simulink model "model"  (R2021a)
settings: Solver=FixedStepAuto  StartTime=0  StopTime=inf  FixedStep=inits.dt  RelTol=1e-3
values from neighbouring files (symbols this model uses):
  inits = load('data.mat')    [main.m]
libraries: aerolibasang x3, shared6dof x1, aerolibatmos2 x1
settings Model: PauseTimes=0.1  Creator=Alper  LastModifiedBy=Alper

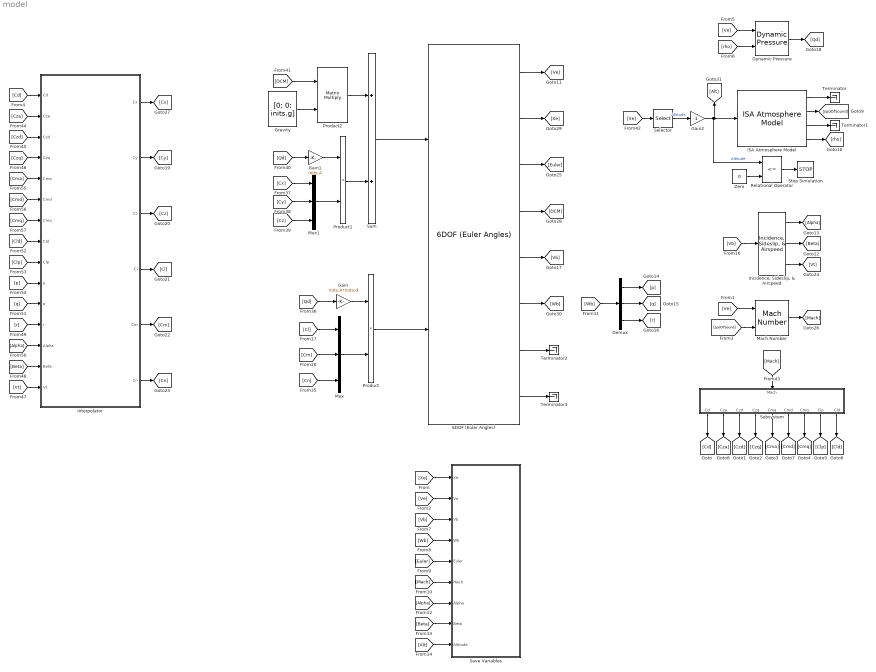
== system model ==
  6DOF (Euler Angles) : shared6dof/6DOF (Euler Angles)  units=Metric (MKS)  mtype=Fixed  rep=Euler Angles  xme_0=[inits.xm inits.ym inits.zm]  Vm_0=[inits.uInit inits.vInit inits.wInit]  eul_0=[inits.phiInit inits.thetaInit inits.psiInit]  pm_0=[inits.pInit inits.qInit inits.rInit]  mass_0=inits.m  mass_e=0.5  mass_f=2.0  inertia=inits.I  inertia_e=eye(3)  inertia_f=2*eye(3)  k_quat=1.0  vre_flag=on  abi_flag=off  aMode=0  xme_statename=''  Vm_statename=''  eul_statename=''  quat_statename=''  pm_statename=''  mass_statename=''
      settings: SourceProductBaseCode=AE,PW,DR,MT,UV,VE
  Demux : Demux  Outputs=3,
  Dynamic Pressure : aerolibasang/Dynamic Pressure
  Gain : Gain  Gain=inits.A*inits.d
  Gain1 : Gain  Gain=inits.A
  Gain2 : Gain  Gain=-1
  Gravity : Constant  Value=[0; 0; inits.g]  VectorParams1D=off
  ISA Atmosphere Model : aerolibatmos2/ISA Atmosphere Model  custom=off  g=9.80665  gamma=1.4  R=287.0531  L=0.0065  h_trop=11000  h_strat=20000  rho0=1.225  P0=101325  T0=288.15  h0=0
  "Incidence, Sideslip, & Airspeed" : aerolibasang/Incidence, Sideslip, & Airspeed
  Interpolator : Subsystem
  Mach Number : aerolibasang/Mach Number
      settings: SourceProductBaseCode=AE
  Mux : Mux  Inputs=3
  Mux1 : Mux  Inputs=3
  Product : Product
  Product1 : Product
  Product2 : Product  Multiplication=Matrix(*)
  Relational Operator : RelationalOperator  Operator=<=  OutDataTypeStr=boolean  RndMeth=Simplest
  Save Variables : Subsystem
  Selector : Selector  InputPortWidth=3  IndexOptions=Index vector (dialog)  Indices=3  OutputSizes=1
  Stop Simulation : Stop
  Subsystem : Subsystem
  Sum : Sum
  Terminator{,1..3} (4 alike) : Terminator
  Zero : Constant  Value=0  OutDataTypeStr=Inherit: Inherit via back propagation
  wires:
  Gain2/1 -> [Alt], ISA Atmosphere Model/1, Relational Operator/1  "Altitude"
  Subsystem/1(Cd) -> [Cd]
  Subsystem/2(Cza) -> [Cza]
  Subsystem/3(Czd) -> [Czd]
  Subsystem/4(Czq) -> [Czq]
  Subsystem/5(Cma) -> [Cma]
  Subsystem/6(Cmd) -> [Cmd]
  Subsystem/7(Cmq) -> [Cmq]
  Subsystem/8(Clp) -> [Clp]
  Subsystem/9(Cld) -> [Cld]
  ISA Atmosphere Model/2 -> [spdOfSound]
  ISA Atmosphere Model/4 -> [rho]
  "Incidence, Sideslip, & Airspeed"/2 -> [Beta]
  "Incidence, Sideslip, & Airspeed"/1 -> [Alpha]
  [Ve] -> Dynamic Pressure/1
  [rho] -> Dynamic Pressure/2
  Demux/1 -> [p]
  Demux/2 -> [q]
  Demux/3 -> [r]
  6DOF (Euler Angles)/1 -> [Ve]
  6DOF (Euler Angles)/5 -> [Vb]
  [Vb] -> "Incidence, Sideslip, & Airspeed"/1
  [spdOfSound] -> Mach Number/2
  [Ve] -> Mach Number/1
  Dynamic Pressure/1 -> [Qd]
  "Incidence, Sideslip, & Airspeed"/3 -> [Vt]
  6DOF (Euler Angles)/3 -> [Euler]
  [Cl] -> Mux/1
  [Cm] -> Mux/2
  [Cn] -> Mux/3
  [Qd] -> Gain/1
  Gain/1 -> Product/1
  Mux/1 -> Product/2
  Product/1 -> 6DOF (Euler Angles)/2
  6DOF (Euler Angles)/4 -> [DCM]
  [Cz] -> Mux1/3
  [Cy] -> Mux1/2
  Product1/1 -> Sum/2
  [Qd] -> Gain1/1
  [Cx] -> Mux1/1
  Gain1/1 -> Product1/1
  Mux1/1 -> Product1/2
  Gravity/1 -> Product2/2
  [DCM] -> Product2/1
  Product2/1 -> Sum/1
  Sum/1 -> 6DOF (Euler Angles)/1
  6DOF (Euler Angles)/2 -> [Xe]
  Zero/1 -> Relational Operator/2
  Relational Operator/1 -> Stop Simulation/1
  Mach Number/1 -> [Mach]
  [Mach] -> Subsystem/1(Mach)
  Interpolator/4(Cl) -> [Cl]
  Interpolator/3(Cz) -> [Cz]
  Interpolator/2(Cy) -> [Cy]
  Interpolator/1(Cx) -> [Cx]
  Interpolator/5(Cm) -> [Cm]
  Interpolator/6(Cn) -> [Cn]
  [Cd] -> Interpolator/1(Cd)
  [Cza] -> Interpolator/2(Cza)
  [Czd] -> Interpolator/3(Czd)
  [Czq] -> Interpolator/4(Czq)
  [Cma] -> Interpolator/5(Cma)
  [Cmd] -> Interpolator/6(Cmd)
  [Cmq] -> Interpolator/7(Cmq)
  [Cld] -> Interpolator/8(Cld)
  [Clp] -> Interpolator/9(Clp)
  [p] -> Interpolator/10(p)
  [q] -> Interpolator/11(q)
  [r] -> Interpolator/12(r)
  [Alpha] -> Interpolator/13(Alpha)
  [Beta] -> Interpolator/14(Beta)
  [Vt] -> Interpolator/15(Vt)
  6DOF (Euler Angles)/6 -> [Wb]
  [Wb] -> Demux/1
  [Xe] -> Save Variables/1(Xe)
  [Ve] -> Save Variables/2(Ve)
  [Vb] -> Save Variables/3(Vb)
  [Wb] -> Save Variables/4(Wb)
  [Euler] -> Save Variables/5(Euler)
  [Mach] -> Save Variables/6(Mach)
  [Alpha] -> Save Variables/7(Alpha)
  [Beta] -> Save Variables/8(Beta)
  [Xe] -> Selector/1
  Selector/1 -> Gain2/1  "Altitude"
  [Alt] -> Save Variables/9(Altitude)
  ISA Atmosphere Model/3 -> Terminator1/1
  ISA Atmosphere Model/1 -> Terminator/1
  6DOF (Euler Angles)/7 -> Terminator2/1
  6DOF (Euler Angles)/8 -> Terminator3/1

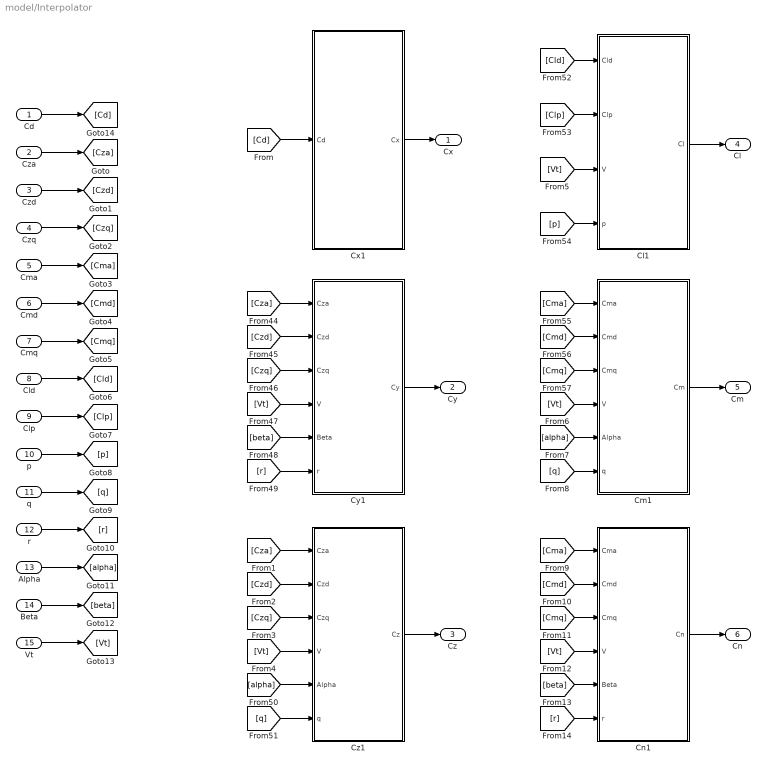
== system model/Interpolator ==
  Cd : Inport
  Cza : Inport  Port=2
  Czd : Inport  Port=3
  Czq : Inport  Port=4
  Cma : Inport  Port=5
  Cmd : Inport  Port=6
  Cmq : Inport  Port=7
  Cld : Inport  Port=8
  Clp : Inport  Port=9
  p : Inport  Port=10
  q : Inport  Port=11
  r : Inport  Port=12
  Alpha : Inport  Port=13
  Beta : Inport  Port=14
  Vt : Inport  Port=15
  Cl1 : Subsystem
  Cm1 : Subsystem
  Cn1 : Subsystem
  Cx1 : Subsystem
  Cy1 : Subsystem
  Cz1 : Subsystem
  Cx : Outport
  Cy : Outport  Port=2
  Cz : Outport  Port=3
  Cl : Outport  Port=4
  Cm : Outport  Port=5
  Cn : Outport  Port=6
  wires:
  Cz1/1(Cz) -> Cz/1
  Cy1/1(Cy) -> Cy/1
  Cl1/1(Cl) -> Cl/1
  Cn1/1(Cn) -> Cn/1
  Cm1/1(Cm) -> Cm/1
  Cza/1 -> [Cza]
  Czd/1 -> [Czd]
  Czq/1 -> [Czq]
  Cma/1 -> [Cma]
  Cmd/1 -> [Cmd]
  Cmq/1 -> [Cmq]
  Cld/1 -> [Cld]
  Clp/1 -> [Clp]
  p/1 -> [p]
  q/1 -> [q]
  r/1 -> [r]
  Alpha/1 -> [alpha]
  Beta/1 -> [beta]
  Vt/1 -> [Vt]
  Cd/1 -> [Cd]
  [Cza] -> Cy1/1(Cza)
  [Czd] -> Cy1/2(Czd)
  [Czq] -> Cy1/3(Czq)
  [Vt] -> Cy1/4(V)
  [beta] -> Cy1/5(Beta)
  [r] -> Cy1/6(r)
  [Cd] -> Cx1/1(Cd)
  [Cza] -> Cz1/1(Cza)
  [Czd] -> Cz1/2(Czd)
  [Czq] -> Cz1/3(Czq)
  [Vt] -> Cz1/4(V)
  [alpha] -> Cz1/5(Alpha)
  [q] -> Cz1/6(q)
  [Clp] -> Cl1/2(Clp)
  [Cld] -> Cl1/1(Cld)
  [Vt] -> Cl1/3(V)
  [p] -> Cl1/4(p)
  [Cma] -> Cm1/1(Cma)
  [Cmd] -> Cm1/2(Cmd)
  [Cmq] -> Cm1/3(Cmq)
  [Vt] -> Cm1/4(V)
  [alpha] -> Cm1/5(Alpha)
  [q] -> Cm1/6(q)
  [Cma] -> Cn1/1(Cma)
  [Cmd] -> Cn1/2(Cmd)
  [Cmq] -> Cn1/3(Cmq)
  [Vt] -> Cn1/4(V)
  [beta] -> Cn1/5(Beta)
  [r] -> Cn1/6(r)
  Cx1/1(Cx) -> Cx/1

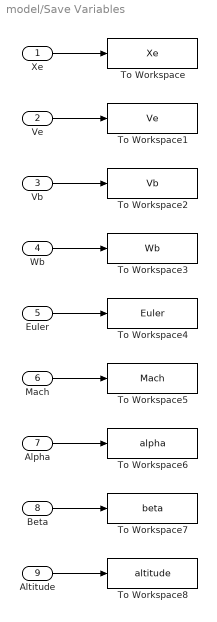
== system model/Save Variables ==
  Xe : Inport
  Ve : Inport  Port=2
  Vb : Inport  Port=3
  Wb : Inport  Port=4
  Euler : Inport  Port=5
  Mach : Inport  Port=6
  Alpha : Inport  Port=7
  Beta : Inport  Port=8
  Altitude : Inport  Port=9
  To Workspace : ToWorkspace  VariableName=Xe  SampleTime=-1
  To Workspace1 : ToWorkspace  VariableName=Ve  SampleTime=-1
  To Workspace2 : ToWorkspace  VariableName=Vb  SampleTime=-1
  To Workspace3 : ToWorkspace  VariableName=Wb  SampleTime=-1
  To Workspace4 : ToWorkspace  VariableName=Euler  SampleTime=-1
  To Workspace5 : ToWorkspace  VariableName=Mach  SampleTime=-1
  To Workspace6 : ToWorkspace  VariableName=alpha  SampleTime=-1
  To Workspace7 : ToWorkspace  VariableName=beta  SampleTime=-1
  To Workspace8 : ToWorkspace  VariableName=altitude  SampleTime=-1
  wires:
  Xe/1 -> To Workspace/1
  Ve/1 -> To Workspace1/1
  Vb/1 -> To Workspace2/1
  Wb/1 -> To Workspace3/1
  Euler/1 -> To Workspace4/1
  Mach/1 -> To Workspace5/1
  Alpha/1 -> To Workspace6/1
  Beta/1 -> To Workspace7/1
  Altitude/1 -> To Workspace8/1

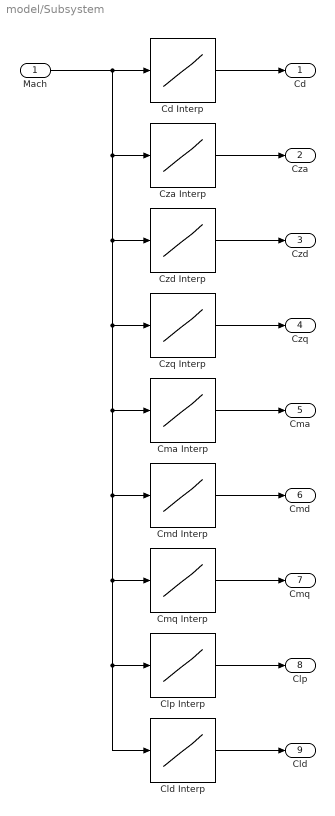
== system model/Subsystem ==
  Mach : Inport
  Cd Interp : Lookup_n-D  NumberOfTableDimensions=1  BreakpointsForDimension1=inits.Machpoints  Table=inits.Cd_data  InternalRulePriority=Speed  RndMeth=Simplest  InputSameDT=on
  Cld Interp : Lookup_n-D  NumberOfTableDimensions=1  BreakpointsForDimension1=inits.Machpoints  Table=inits.Cld_data  InternalRulePriority=Speed  RndMeth=Simplest  InputSameDT=on
  Clp Interp : Lookup_n-D  NumberOfTableDimensions=1  BreakpointsForDimension1=inits.Machpoints  Table=inits.Clp_data  InternalRulePriority=Speed  RndMeth=Simplest  InputSameDT=on
  Cma Interp : Lookup_n-D  NumberOfTableDimensions=1  BreakpointsForDimension1=inits.Machpoints  Table=inits.Cma_data  InternalRulePriority=Speed  RndMeth=Simplest  InputSameDT=on
  Cmd Interp : Lookup_n-D  NumberOfTableDimensions=1  BreakpointsForDimension1=inits.Machpoints  Table=inits.Cmd_data  InternalRulePriority=Speed  RndMeth=Simplest  InputSameDT=on
  Cmq Interp : Lookup_n-D  NumberOfTableDimensions=1  BreakpointsForDimension1=inits.Machpoints  Table=inits.Cmq_data  InternalRulePriority=Speed  RndMeth=Simplest  InputSameDT=on
  Cza Interp : Lookup_n-D  NumberOfTableDimensions=1  BreakpointsForDimension1=inits.Machpoints  Table=inits.Cza_data  InternalRulePriority=Speed  RndMeth=Simplest  InputSameDT=on
  Czd Interp : Lookup_n-D  NumberOfTableDimensions=1  BreakpointsForDimension1=inits.Machpoints  Table=inits.Czd_data  InternalRulePriority=Speed  RndMeth=Simplest  InputSameDT=on
  Czq Interp : Lookup_n-D  NumberOfTableDimensions=1  BreakpointsForDimension1=inits.Machpoints  Table=inits.Czq_data  InternalRulePriority=Speed  RndMeth=Simplest  InputSameDT=on
  Cd : Outport
  Cza : Outport  Port=2
  Czd : Outport  Port=3
  Czq : Outport  Port=4
  Cma : Outport  Port=5
  Cmd : Outport  Port=6
  Cmq : Outport  Port=7
  Clp : Outport  Port=8
  Cld : Outport  Port=9
  wires:
  Cmd Interp/1 -> Cmd/1
  Cd Interp/1 -> Cd/1
  Clp Interp/1 -> Clp/1
  Cld Interp/1 -> Cld/1
  Czd Interp/1 -> Czd/1
  Czq Interp/1 -> Czq/1
  Mach/1 -> Cza Interp/1, Czd Interp/1, Czq Interp/1, Cma Interp/1, Cmd Interp/1, Cmq Interp/1, Clp Interp/1, Cld Interp/1, Cd Interp/1
  Cmq Interp/1 -> Cmq/1
  Cza Interp/1 -> Cza/1
  Cma Interp/1 -> Cma/1

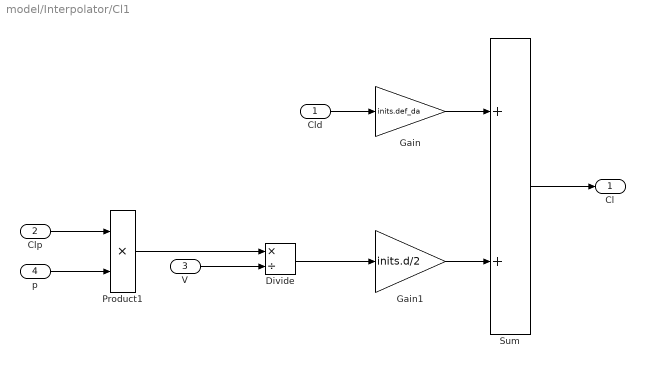
== system model/Interpolator/Cl1 ==
  Cld : Inport
  Clp : Inport  Port=2
  V : Inport  Port=3
  p : Inport  Port=4
  Divide : Product  Inputs=*/
  Gain : Gain  Gain=inits.def_da
  Gain1 : Gain  Gain=inits.d/2
  Product1 : Product
  Sum : Sum
  Cl : Outport
  wires:
  Cld/1 -> Gain/1
  Clp/1 -> Product1/1
  p/1 -> Product1/2
  Product1/1 -> Divide/1
  V/1 -> Divide/2
  Divide/1 -> Gain1/1
  Gain1/1 -> Sum/2
  Sum/1 -> Cl/1
  Gain/1 -> Sum/1

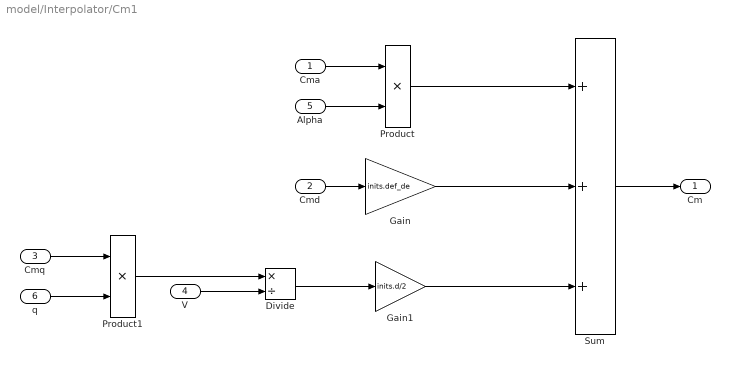
== system model/Interpolator/Cm1 ==
  Cma : Inport
  Cmd : Inport  Port=2
  Cmq : Inport  Port=3
  V : Inport  Port=4
  Alpha : Inport  Port=5
  q : Inport  Port=6
  Divide : Product  Inputs=*/
  Gain : Gain  Gain=inits.def_de
  Gain1 : Gain  Gain=inits.d/2
  Product : Product
  Product1 : Product
  Sum : Sum  Inputs=+++
  Cm : Outport
  wires:
  Cma/1 -> Product/1
  Alpha/1 -> Product/2
  Cmd/1 -> Gain/1
  Cmq/1 -> Product1/1
  q/1 -> Product1/2
  Product1/1 -> Divide/1
  V/1 -> Divide/2
  Divide/1 -> Gain1/1
  Product/1 -> Sum/1
  Gain/1 -> Sum/2
  Gain1/1 -> Sum/3
  Sum/1 -> Cm/1

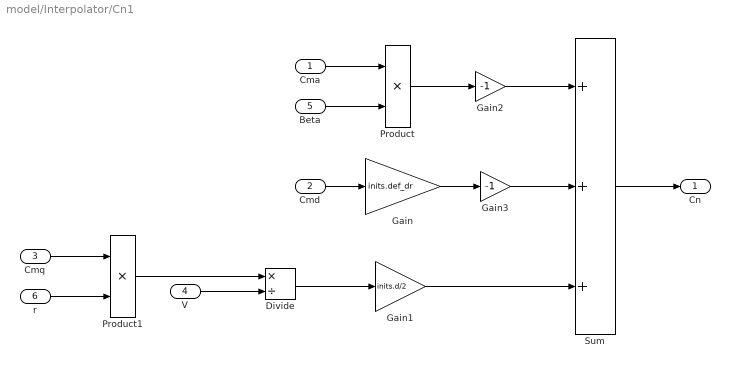
== system model/Interpolator/Cn1 ==
  Cma : Inport
  Cmd : Inport  Port=2
  Cmq : Inport  Port=3
  V : Inport  Port=4
  Beta : Inport  Port=5
  r : Inport  Port=6
  Divide : Product  Inputs=*/
  Gain : Gain  Gain=inits.def_dr
  Gain1 : Gain  Gain=inits.d/2
  Gain2 : Gain  Gain=-1
  Gain3 : Gain  Gain=-1
  Product : Product
  Product1 : Product
  Sum : Sum  Inputs=+++
  Cn : Outport
  wires:
  Cma/1 -> Product/1
  Beta/1 -> Product/2
  Cmd/1 -> Gain/1
  Cmq/1 -> Product1/1
  r/1 -> Product1/2
  Product1/1 -> Divide/1
  V/1 -> Divide/2
  Divide/1 -> Gain1/1
  Gain1/1 -> Sum/3
  Sum/1 -> Cn/1
  Product/1 -> Gain2/1
  Gain2/1 -> Sum/1
  Gain/1 -> Gain3/1
  Gain3/1 -> Sum/2

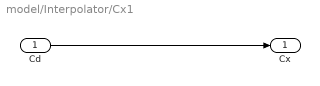
== system model/Interpolator/Cx1 ==
  Cd : Inport
  Cx : Outport
  wires:
  Cd/1 -> Cx/1

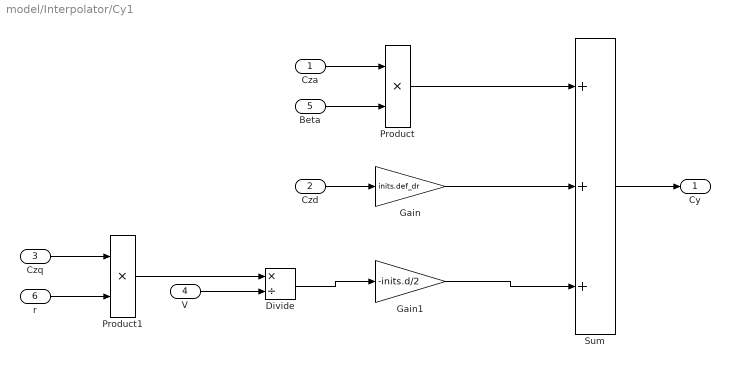
== system model/Interpolator/Cy1 ==
  Cza : Inport
  Czd : Inport  Port=2
  Czq : Inport  Port=3
  V : Inport  Port=4
  Beta : Inport  Port=5
  r : Inport  Port=6
  Divide : Product  Inputs=*/
  Gain : Gain  Gain=inits.def_dr
  Gain1 : Gain  Gain=-inits.d/2
  Product : Product
  Product1 : Product
  Sum : Sum  Inputs=+++
  Cy : Outport
  wires:
  Cza/1 -> Product/1
  Beta/1 -> Product/2
  Czd/1 -> Gain/1
  Czq/1 -> Product1/1
  r/1 -> Product1/2
  Product1/1 -> Divide/1
  V/1 -> Divide/2
  Divide/1 -> Gain1/1
  Product/1 -> Sum/1
  Gain/1 -> Sum/2
  Gain1/1 -> Sum/3
  Sum/1 -> Cy/1

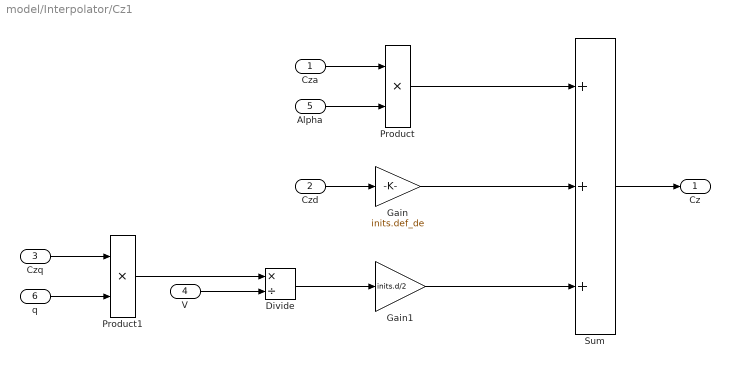
== system model/Interpolator/Cz1 ==
  Cza : Inport
  Czd : Inport  Port=2
  Czq : Inport  Port=3
  V : Inport  Port=4
  Alpha : Inport  Port=5
  q : Inport  Port=6
  Divide : Product  Inputs=*/
  Gain : Gain  Gain=inits.def_de
  Gain1 : Gain  Gain=inits.d/2
  Product : Product
  Product1 : Product
  Sum : Sum  Inputs=+++
  Cz : Outport
  wires:
  Cza/1 -> Product/1
  Alpha/1 -> Product/2
  Czd/1 -> Gain/1
  Czq/1 -> Product1/1
  q/1 -> Product1/2
  Product1/1 -> Divide/1
  V/1 -> Divide/2
  Divide/1 -> Gain1/1
  Product/1 -> Sum/1
  Gain/1 -> Sum/2
  Gain1/1 -> Sum/3
  Sum/1 -> Cz/1
